simulink model "excercise"  (R2019b)
settings: Solver=FixedStepAuto  StartTime=0.0  StopTime=10.0  FixedStep=1/200  RelTol=1e-3
settings Model: Creator=omiks  LastModifiedBy=omiks

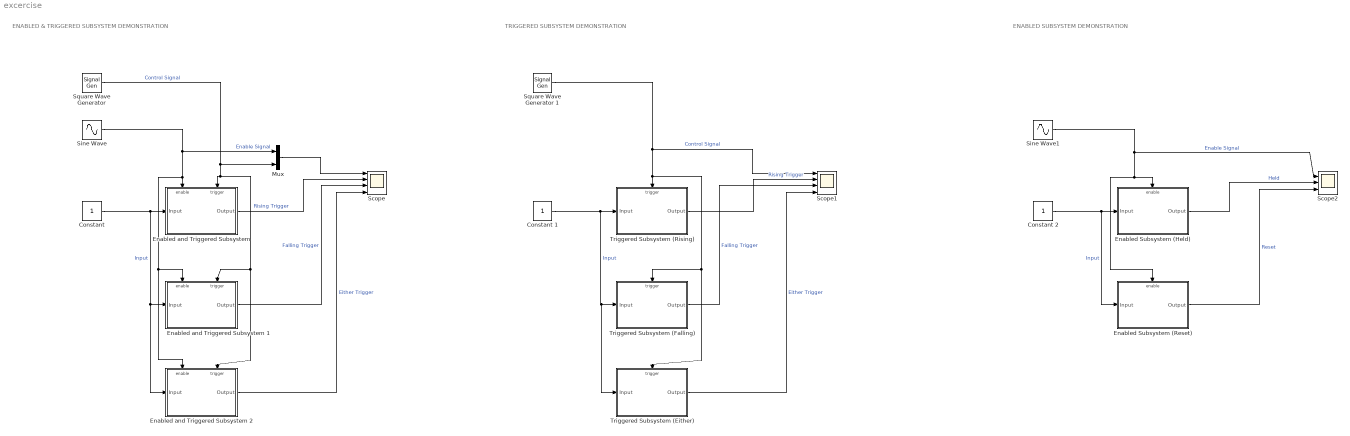
== system excercise ==
  note: ENABLED & TRIGGERED SUBSYSTEM DEMONSTRATION
  note: TRIGGERED SUBSYSTEM DEMONSTRATION
  note: ENABLED SUBSYSTEM DEMONSTRATION
  " Triggered Subsystem (Either)" : Subsystem  TreatAsAtomicUnit=on
  " Triggered Subsystem (Falling) " : Subsystem  TreatAsAtomicUnit=on
  " Triggered Subsystem (Rising)" : Subsystem  TreatAsAtomicUnit=on
  "Constant " : Constant
  Constant 1 : Constant
  Constant 2 : Constant
  "Enabled Subsystem (Held) " : Subsystem  TreatAsAtomicUnit=on
  "Enabled Subsystem (Reset) " : Subsystem  TreatAsAtomicUnit=on
  "Enabled and Triggered Subsystem " : Subsystem  TreatAsAtomicUnit=on
  Enabled and Triggered Subsystem 1 : Subsystem  TreatAsAtomicUnit=on
  Enabled and Triggered Subsystem 2 : Subsystem  TreatAsAtomicUnit=on
  Mux : Mux  Inputs=2
  Scope : Scope  NumInputPorts=4
  Scope1 : Scope  NumInputPorts=4
  Scope2 : Scope  NumInputPorts=3
  Sine Wave : Sin  SineType=Sample based  Samples=600  SampleTime=1/200
  Sine Wave1 : Sin  SineType=Sample based  Samples=600  SampleTime=1/200
  "Square Wave Generator " : SignalGenerator  WaveForm=square  Frequency=7  Units=rad/sec
  Square Wave Generator 1 : SignalGenerator  WaveForm=square  Frequency=7  Units=rad/sec
  wires:
  "Square Wave Generator "/1 -> Mux/2, Enabled and Triggered Subsystem 2/Trigger, Enabled and Triggered Subsystem 1/Trigger, "Enabled and Triggered Subsystem "/Trigger  "Control Signal"
  Sine Wave/1 -> Mux/1, Enabled and Triggered Subsystem 1/Enable, Enabled and Triggered Subsystem 2/Enable, "Enabled and Triggered Subsystem "/Enable  "Enable Signal"
  "Enabled and Triggered Subsystem "/1("Output ") -> Scope/2  "Rising Trigger"
  "Constant "/1 -> Enabled and Triggered Subsystem 2/1(Input), Enabled and Triggered Subsystem 1/1(Input), "Enabled and Triggered Subsystem "/1(Input)  "Input"
  Mux/1 -> Scope/1
  Enabled and Triggered Subsystem 1/1("Output ") -> Scope/3  "Falling Trigger"
  Enabled and Triggered Subsystem 2/1("Output ") -> Scope/4  "Either Trigger"
  Constant 1/1 -> " Triggered Subsystem (Either)"/1(Input), " Triggered Subsystem (Falling) "/1(Input), " Triggered Subsystem (Rising)"/1(Input)  "Input"
  " Triggered Subsystem (Falling) "/1("Output ") -> Scope1/3  "Falling Trigger"
  " Triggered Subsystem (Rising)"/1("Output ") -> Scope1/2  "Rising Trigger"
  " Triggered Subsystem (Either)"/1("Output ") -> Scope1/4  "Either Trigger"
  Square Wave Generator 1/1 -> " Triggered Subsystem (Either)"/Trigger, " Triggered Subsystem (Falling) "/Trigger, " Triggered Subsystem (Rising)"/Trigger, Scope1/1  "Control Signal"
  Constant 2/1 -> "Enabled Subsystem (Reset) "/1(Input), "Enabled Subsystem (Held) "/1(Input)  "Input"
  Sine Wave1/1 -> "Enabled Subsystem (Reset) "/Enable, "Enabled Subsystem (Held) "/Enable, Scope2/1  "Enable Signal"
  "Enabled Subsystem (Reset) "/1("Output ") -> Scope2/3  "Reset"
  "Enabled Subsystem (Held) "/1("Output ") -> Scope2/2  "Held"

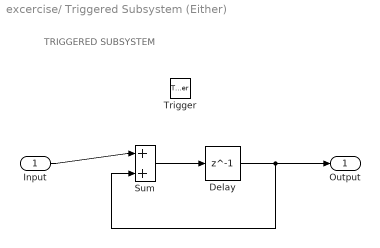
== system excercise/ Triggered Subsystem (Either) ==
  note: TRIGGERED SUBSYSTEM
  Input : Inport
  Trigger : TriggerPort  TriggerType=either  VariantControl=Variant
  Delay : Delay  DelayLength=1
  Sum : Sum  Inputs=|++
  "Output " : Outport
  wires:
  Input/1 -> Sum/1
  Sum/1 -> Delay/1
  Delay/1 -> "Output "/1, Sum/2

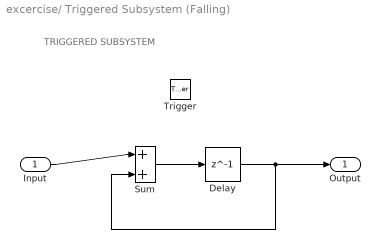
== system excercise/ Triggered Subsystem (Falling)  ==
  note: TRIGGERED SUBSYSTEM
  Input : Inport
  Trigger : TriggerPort  TriggerType=falling  VariantControl=Variant
  Delay : Delay  DelayLength=1
  Sum : Sum  Inputs=|++
  "Output " : Outport
  wires:
  Input/1 -> Sum/1
  Sum/1 -> Delay/1
  Delay/1 -> "Output "/1, Sum/2

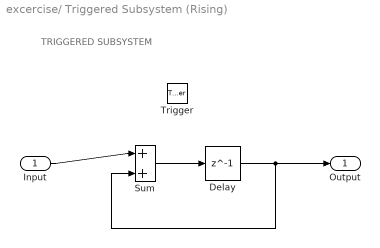
== system excercise/ Triggered Subsystem (Rising) ==
  note: TRIGGERED SUBSYSTEM
  Input : Inport
  Trigger : TriggerPort  VariantControl=Variant  PortDimensions=1
  Delay : Delay  DelayLength=1
  Sum : Sum  Inputs=|++
  "Output " : Outport
  wires:
  Input/1 -> Sum/1
  Sum/1 -> Delay/1
  Delay/1 -> "Output "/1, Sum/2

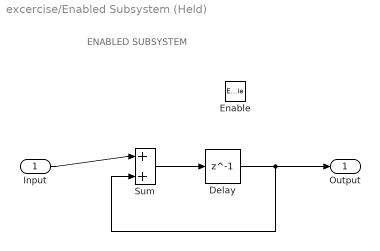
== system excercise/Enabled Subsystem (Held)  ==
  note: ENABLED SUBSYSTEM
  Input : Inport
  Enable : EnablePort
  Delay : Delay  DelayLength=1
  Sum : Sum  Inputs=|++
  "Output " : Outport
  wires:
  Input/1 -> Sum/1
  Sum/1 -> Delay/1
  Delay/1 -> "Output "/1, Sum/2

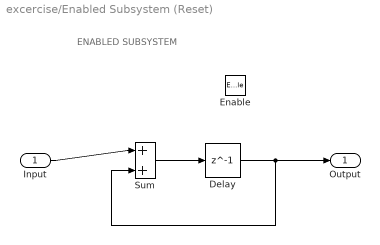
== system excercise/Enabled Subsystem (Reset)  ==
  note: ENABLED SUBSYSTEM
  Input : Inport
  Enable : EnablePort  StatesWhenEnabling=reset
  Delay : Delay  DelayLength=1
  Sum : Sum  Inputs=|++
  "Output " : Outport
  wires:
  Input/1 -> Sum/1
  Sum/1 -> Delay/1
  Delay/1 -> "Output "/1, Sum/2

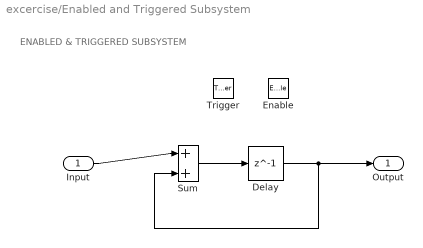
== system excercise/Enabled and Triggered Subsystem  ==
  note: ENABLED & TRIGGERED SUBSYSTEM
  Input : Inport
  Enable : EnablePort  StatesWhenEnabling=reset
  Trigger : TriggerPort  VariantControl=Variant
  Delay : Delay  DelayLength=1
  Sum : Sum  Inputs=|++
  "Output " : Outport
  wires:
  Input/1 -> Sum/1
  Sum/1 -> Delay/1
  Delay/1 -> "Output "/1, Sum/2

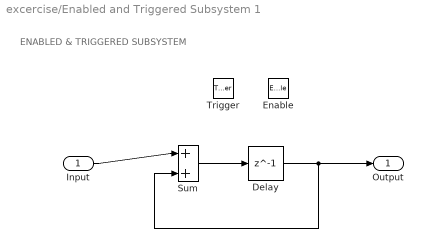
== system excercise/Enabled and Triggered Subsystem 1 ==
  note: ENABLED & TRIGGERED SUBSYSTEM
  Input : Inport
  Enable : EnablePort  StatesWhenEnabling=reset
  Trigger : TriggerPort  TriggerType=falling  VariantControl=Variant
  Delay : Delay  DelayLength=1
  Sum : Sum  Inputs=|++
  "Output " : Outport
  wires:
  Input/1 -> Sum/1
  Sum/1 -> Delay/1
  Delay/1 -> "Output "/1, Sum/2

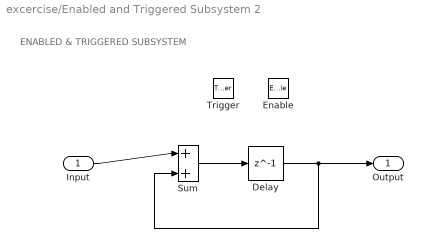
== system excercise/Enabled and Triggered Subsystem 2 ==
  note: ENABLED & TRIGGERED SUBSYSTEM
  Input : Inport
  Enable : EnablePort  StatesWhenEnabling=reset
  Trigger : TriggerPort  TriggerType=either  VariantControl=Variant
  Delay : Delay  DelayLength=1
  Sum : Sum  Inputs=|++
  "Output " : Outport
  wires:
  Input/1 -> Sum/1
  Sum/1 -> Delay/1
  Delay/1 -> "Output "/1, Sum/2
